simulink subsystem "Actuator_Thruster"  (R2025a)
settings: Solver=VariableStepAuto  StartTime=0.0  StopTime=10.0  RelTol=1e-3
undefined symbols (not defined in the file): IAU, WMM2025
libraries: aerolibtransform2 x1, aerolibgravity2 x1
settings Model: Creator=Jackt  LastModifiedBy=Jackt

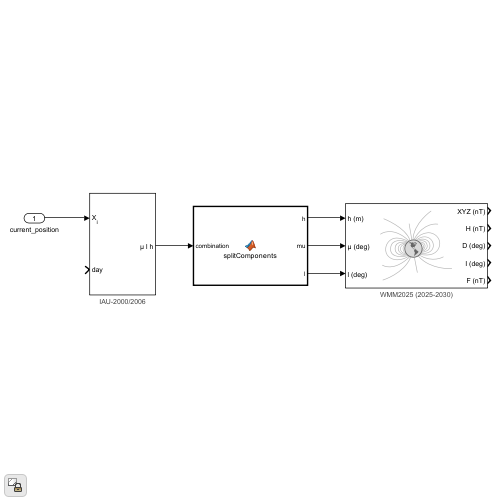
[thumbnail: Simulink's stored preview of the top-level diagram]
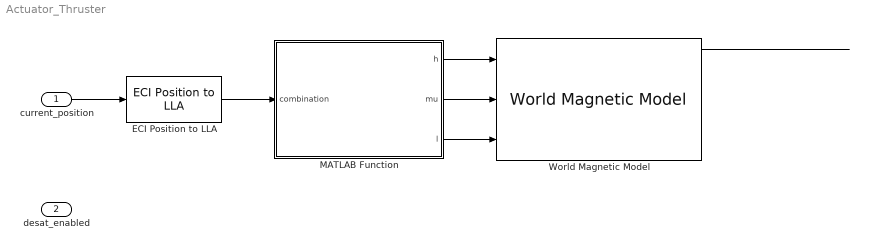
== system Actuator_Thruster ==
  current_position : Inport
  desat_enabled : Inport  Port=2
  ECI Position to LLA : aerolibtransform2/ECI Position to LLA  red=IAU-2000/2006  year=2026  month=January  day=1  hour=0  min=0  sec=0  deltaT=None  errorflag=Error  extraparamflag=off  eunits=Metric (MKS)  earthmodel=WGS84  flat=1/298.257223563  eqradius=6378137
      settings: AttributesFormatString=%<red>
  MATLAB Function : MATLAB Function  TreatAsAtomicUnit=on
  World Magnetic Model : aerolibgravity2/World Magnetic Model  model=WMM2025 (2025-2030)  customFile='WMM2025.COF'  units=Metric (MKS)  time_in=off  month=January  day=1  year=2025  action=Error  h_out=on  dec_out=on  inc_out=on  ti_out=on
  wires:
  current_position/1 -> ECI Position to LLA/1
  ECI Position to LLA/1 -> MATLAB Function/1(combination)
  MATLAB Function/1(h) -> World Magnetic Model/1
  MATLAB Function/2(mu) -> World Magnetic Model/2
  MATLAB Function/3(l) -> World Magnetic Model/3
  World Magnetic Model/1 -> ?

== matlab function Actuator_Thruster/MATLAB Function ==
  data: combination input; h output; mu output; l output
function [h, mu, l] = splitComponents(combination)
h = combination(3);
mu = combination(1);
l = combination(2);
